simulink model "roboticArm"  (R2021a)
settings: Solver=FixedStepDiscrete  StartTime=0.0  StopTime=inf  FixedStep=0.001  RelTol=1e-3  EnableMultiTasking=on
PreLoadFcn:
  | set_param(gcs, 'RTWSystemTargetFile', 'franka_emika_panda.tlc');%
  | %initRoboticArm();
values from neighbouring files (symbols this model uses):
  amp = 0.05*100    (= 5)    [initRoboticArm.m]    (also in initRoboticArm2.m = 0.5)
  dof = 1    [initRoboticArm.m]    (also in initRoboticArm2.m)
  init_delay = 10    [initRoboticArm.m]    (also in initRoboticArm2.m)
  Kd_matr = zeros(6)    [initRoboticArm.m]    (also in init_roboticArm_loadCell.m = diag([0.00;0;0.003;0.0001;0.00;0.0001]); zeroForce2.mat = [0 0 0 0 0 0 0 0 0 0 0 0 ... (36 elements, 6x6)])
  Ki_matr = zeros(6)    [initRoboticArm.m]    (also in init_roboticArm_loadCell.m = diag([10;100;10;30;10;2]); zeroForce2.mat = [10 0 0 0 0 0 0 100 0 0 0 0 ... (36 elements, 6x6)])
  Kp_matr = zeros(6)    [initRoboticArm.m]    (also in init_roboticArm_loadCell.m = diag([0.3;0.1;0.2;0.05;0.3;0.2]); zeroForce2.mat = [0.3 0 0 0 0 0 0 0.1 0 0 0 0 ... (36 elements, 6x6)])
  scaled_array = zeros(round((chirp_duration+10)*1./dt-1)+1,7)    [initRoboticArm.m]    (also in init_roboticArm_loadCell.m = [scaled_array(:,1) zeros(length(scaled_array),6)]; scaled_array_oc5.mat = [0 0.0141421356237 0.0282842712475 0.0424264068712 0.0565685; zeroForce2.mat = [0 0.0141421356237 0.0282842712475 0.0424264068712 0.0565685)
  tuning_signal = 2    [initRoboticArm.m]    (also in initRoboticArm2.m = 4)
undefined symbols (not defined in the file or in its folder): DiscIntNeverNeededParam
libraries: spsSampleandHoldLib x12, franka_simulink_library x5, simulink x3, etargetslib x1, dspnetwork x1
settings Model: ExtModeTrigDuration=10000  Creator=vasi_ko  LastModifiedBy=host
settings SolverCC: AlgebraicLoopSolver=TrustRegion
settings DataIOCC: SaveFormat=Array  ReturnWorkspaceOutputs=off
settings OptimizationCC: DefaultParameterBehavior=Inlined  EnhancedBackFolding=on  PassReuseOutputArgsThreshold=0  OptimizeBlockOrder=speed  DifferentSizesBufferReuse=on  OptimizationCustomize=off
settings DebuggingCC: SolverPrmCheckMsg=warning  ParameterTunabilityLossMsg=error  SFUnexpectedBacktrackingDiag=warning  SFNoUnconditionalDefaultTransitionDiag=warning  SFExecutionAtInitializationDiag=none  SFMachineParentedDataDiag=warning  ArithmeticOperatorsInVariantConditions=warning
settings HardwareCC: ProdBitPerLong=64  ProdHWDeviceType=Intel->x86-64 (Linux 64)
settings ModelReferenceCC: PropagateSignalLabelsOutOfModel=off
settings SFSimCC: SimUseLocalCustomCode=off  MATLABDynamicMemAlloc=off  CustomCodeUndefinedFunction=UseInterfaceOnly  SimTargetLang=C++
settings RTWCC: Description=Generic Real-Time Target  SystemTargetFile=franka_emika_panda.tlc  RTWVerbose=off  RTWUseLocalCustomCode=off  Toolchain=Franka Simulink | gmake (64-bit linux)  BuildConfiguration=Faster Runs  TargetLang=C++
settings CodeAppCC: ForceParamTrailComments=on  OperatorAnnotations=on
settings STFCustomTargetCC: TargetLangStandard=C99 (ISO)  ModelReferenceCompliant=off  MatFileLogging=on  SystemTargetFile=franka_emika_panda.tlc
settings GRTTargetCC: ModelReferenceCompliant=off  ParMdlRefBuildCompliant=off  CompOptLevelCompliant=off  ConcurrentExecutionCompliant=off  CombineOutputUpdateFcns=off  CPPClassGenCompliant=off  GRTInterface=on  ExtModeStaticAlloc=on  ExtModeTransport=1  ExtModeMexFile=ext_xcp  ExtModeIntrfLevel=Level2 - Open
settings ConfigComp: CovMetricSettings=dw  CovSaveCumulativeToWorkspaceVar=on  CovSaveSingleToWorkspaceVar=on  CovExternalEMLEnable=off  CovSFcnEnable=off

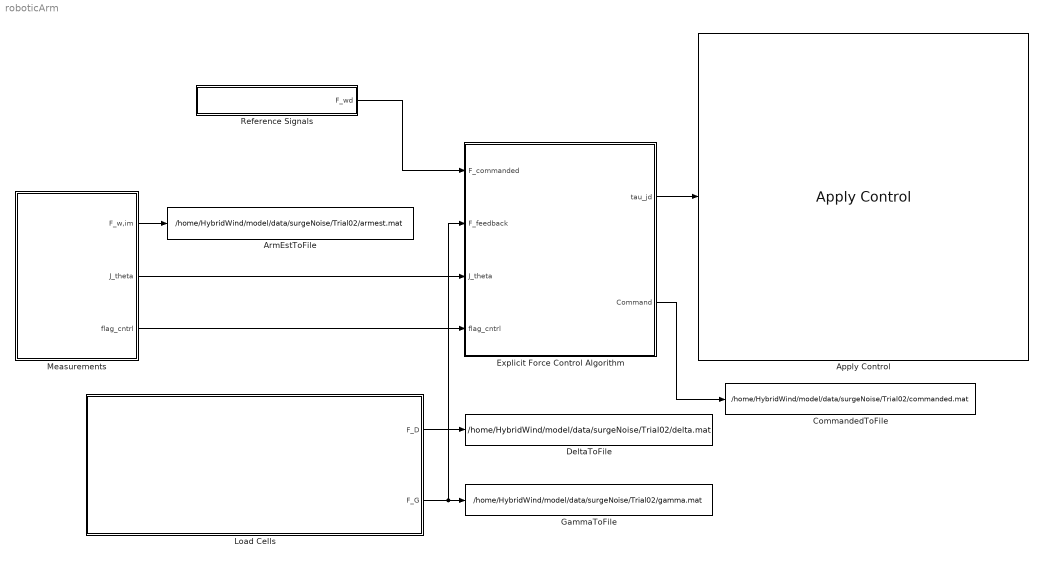
== system roboticArm ==
  Apply Control : franka_simulink_library/Apply Control  robot_ip=robot_ip  gripper_attached=off  control_mode=Torque Control  controller_choice=Joint Impedance Controller  elbow_control=on  collision_thresholds=100*ones(1,52)  joint_impedance=joint_impedance  cartesian_impedance=cartesian_impedance  load_inertia=load_inertia  EE_T_K=EE_T_K  init_joint_configuration_req=off  init_joint_configuration=[0.00392584915725334;-0.104076810189763;0.0404703493577216;-2.7334242600631;0.0113035300040543;2.63364770337236;0.372162046953987]
      settings: SourceProductName=Franka Emika
  ArmEstToFile : ToFile  Filename=/home/HybridWind/model/data/surgeNoise/Trial02/armest.mat  MatrixName=armest
  CommandedToFile : ToFile  Filename=/home/HybridWind/model/data/surgeNoise/Trial02/commanded.mat  MatrixName=commanded
  DeltaToFile : ToFile  Filename=/home/HybridWind/model/data/surgeNoise/Trial02/delta.mat  MatrixName=delta
  Explicit Force Control Algorithm : Subsystem
  GammaToFile : ToFile  Filename=/home/HybridWind/model/data/surgeNoise/Trial02/gamma.mat  MatrixName=gamma
  Load Cells : Subsystem
  Measurements : Subsystem
  Reference Signals : Subsystem
  wires:
  Measurements/3(flag_cntrl) -> Explicit Force Control Algorithm/4(flag_cntrl)
  Load Cells/2(F_G) -> Explicit Force Control Algorithm/2(F_feedback), GammaToFile/1
  Explicit Force Control Algorithm/1(tau_jd) -> Apply Control/1
  Reference Signals/1(F_wd) -> Explicit Force Control Algorithm/1(F_commanded)
  Measurements/2(J_theta) -> Explicit Force Control Algorithm/3(J_theta)
  Measurements/1(F_w,im) -> ArmEstToFile/1
  Explicit Force Control Algorithm/2(Command) -> CommandedToFile/1
  Load Cells/1(F_D) -> DeltaToFile/1

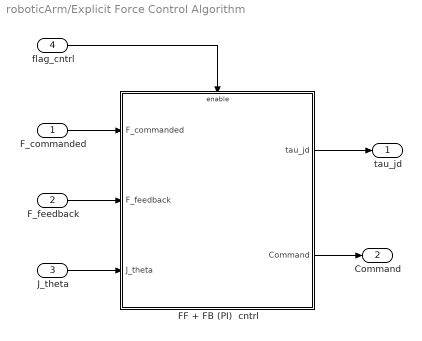
== system roboticArm/Explicit Force Control Algorithm ==
  F_commanded : Inport
  F_feedback : Inport  Port=2
  J_theta : Inport  Port=3
  flag_cntrl : Inport  Port=4
  FF + FB (PI)  cntrl : Subsystem
  tau_jd : Outport
  Command : Outport  Port=2
  wires:
  F_commanded/1 -> FF + FB (PI)  cntrl/1(F_commanded)
  F_feedback/1 -> FF + FB (PI)  cntrl/2(F_feedback)
  J_theta/1 -> FF + FB (PI)  cntrl/3(J_theta)
  FF + FB (PI)  cntrl/1(tau_jd) -> tau_jd/1
  flag_cntrl/1 -> FF + FB (PI)  cntrl/Enable
  FF + FB (PI)  cntrl/2(Command) -> Command/1

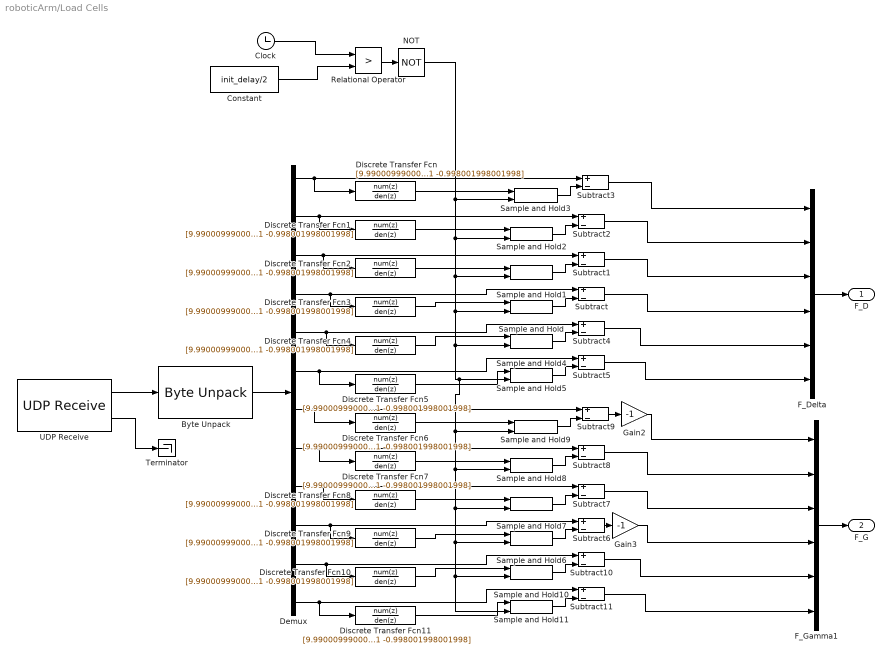
== system roboticArm/Load Cells ==
  Byte Unpack : etargetslib/Byte Unpack  dimensions={[12]}  datatypes={'double'}  byteAlign=1
  Clock : Clock
  Constant : Constant  Value=init_delay/2
  Demux : Demux  Outputs=12
  Discrete Transfer Fcn{,1..11} (12 alike) : DiscreteTransferFcn  Numerator=[9.990009990009990e-04 9.990009990009990e-04]  Denominator=[1 -0.998001998001998]
  F_Delta : Mux  Inputs=6
  F_Gamma1 : Mux  Inputs=6
  Gain2 : Gain  Gain=-1
  Gain3 : Gain  Gain=-1
  NOT : Logic  Operator=NOT  IconShape=distinctive  AllPortsSameDT=off  OutDataTypeStr=boolean
  Relational Operator : RelationalOperator  Operator=>  OutDataTypeStr=boolean  RndMeth=Simplest
  Sample and Hold{,1..11} (12 alike) : spsSampleandHoldLib/Sample and Hold  ic=0  Ts=0
      settings: SourceProductBaseCode=PS
  Subtract{,1..11} (12 alike) : Sum  Inputs=+-
  Terminator : Terminator
  UDP Receive : dspnetwork/UDP Receive  localURL='0.0.0.0'  localPort=8002  remoteURL='10.10.10.15'  remotePort=-1  recvBufferSize=8192  dims=96  signalDatatype=uint8  isComplex=off  isVarSize=off  showBlockingTime=on  blockingTime=inf  sampletime=0.001  blockPlatform=HOST
  F_D : Outport
  F_G : Outport  Port=2
  wires:
  UDP Receive/1 -> Byte Unpack/1
  Constant/1 -> Relational Operator/2
  Relational Operator/1 -> NOT/1
  Sample and Hold/1 -> Subtract/2
  UDP Receive/2 -> Terminator/1
  Demux/4 -> Discrete Transfer Fcn3/1, Subtract/1
  Clock/1 -> Relational Operator/1
  Byte Unpack/1 -> Demux/1
  Demux/3 -> Discrete Transfer Fcn2/1, Subtract1/1
  Sample and Hold1/1 -> Subtract1/2
  Subtract1/1 -> F_Delta/3
  Subtract2/1 -> F_Delta/2
  Sample and Hold2/1 -> Subtract2/2
  Demux/2 -> Discrete Transfer Fcn1/1, Subtract2/1
  Sample and Hold3/1 -> Subtract3/2
  Subtract4/1 -> F_Delta/5
  Sample and Hold4/1 -> Subtract4/2
  Demux/5 -> Discrete Transfer Fcn4/1, Subtract4/1
  Demux/6 -> Discrete Transfer Fcn5/1, Subtract5/1
  Sample and Hold5/1 -> Subtract5/2
  Subtract5/1 -> F_Delta/6
  Subtract3/1 -> F_Delta/1
  Subtract/1 -> F_Delta/4
  F_Delta/1 -> F_D/1
  Demux/1 -> Discrete Transfer Fcn/1, Subtract3/1
  Discrete Transfer Fcn/1 -> Sample and Hold3/1
  Discrete Transfer Fcn1/1 -> Sample and Hold2/1
  Discrete Transfer Fcn2/1 -> Sample and Hold1/1
  Discrete Transfer Fcn3/1 -> Sample and Hold/1
  Discrete Transfer Fcn4/1 -> Sample and Hold4/1
  Discrete Transfer Fcn5/1 -> Sample and Hold5/1
  Discrete Transfer Fcn11/1 -> Sample and Hold11/1
  Discrete Transfer Fcn10/1 -> Sample and Hold10/1
  Discrete Transfer Fcn9/1 -> Sample and Hold6/1
  Discrete Transfer Fcn8/1 -> Sample and Hold7/1
  Discrete Transfer Fcn7/1 -> Sample and Hold8/1
  Discrete Transfer Fcn6/1 -> Sample and Hold9/1
  Demux/7 -> Subtract9/1, Discrete Transfer Fcn6/1
  F_Gamma1/1 -> F_G/1
  Gain3/1 -> F_Gamma1/4
  Gain2/1 -> F_Gamma1/1
  Subtract11/1 -> F_Gamma1/6
  Sample and Hold11/1 -> Subtract11/2
  NOT/1 -> Sample and Hold3/2, Sample and Hold2/2, Sample and Hold1/2, Sample and Hold6/2, Sample and Hold10/2, Sample and Hold11/2, Sample and Hold7/2, Sample and Hold8/2, Sample and Hold9/2, Sample and Hold5/2, Sample and Hold4/2, Sample and Hold/2
  Demux/12 -> Subtract11/1, Discrete Transfer Fcn11/1
  Demux/11 -> Subtract10/1, Discrete Transfer Fcn10/1
  Sample and Hold10/1 -> Subtract10/2
  Subtract10/1 -> F_Gamma1/5
  Subtract9/1 -> Gain2/1
  Sample and Hold9/1 -> Subtract9/2
  Demux/8 -> Subtract8/1, Discrete Transfer Fcn7/1
  Sample and Hold8/1 -> Subtract8/2
  Subtract8/1 -> F_Gamma1/2
  Subtract7/1 -> F_Gamma1/3
  Sample and Hold7/1 -> Subtract7/2
  Demux/9 -> Subtract7/1, Discrete Transfer Fcn8/1
  Demux/10 -> Subtract6/1, Discrete Transfer Fcn9/1
  Sample and Hold6/1 -> Subtract6/2
  Subtract6/1 -> Gain3/1

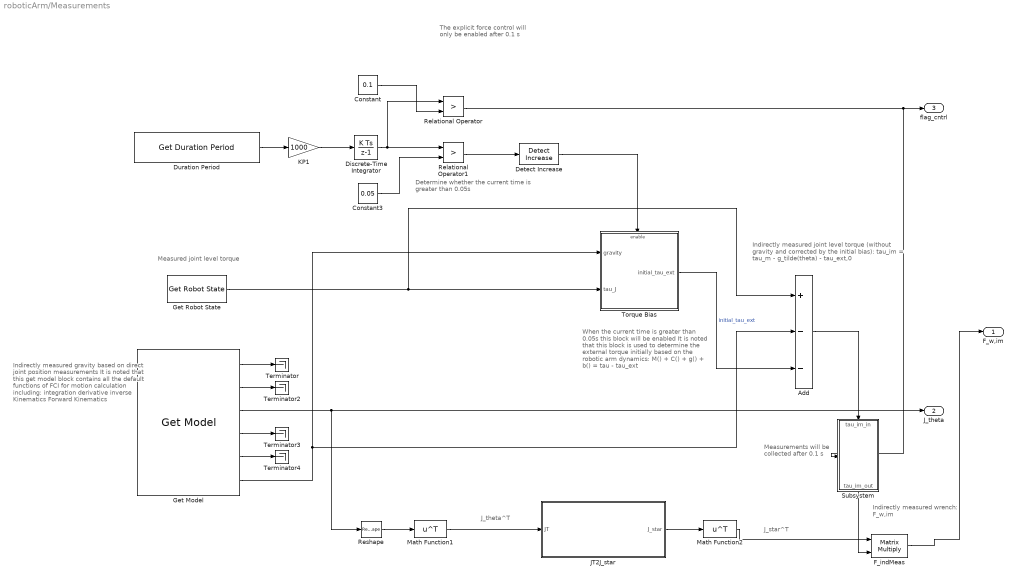
== system roboticArm/Measurements ==
  note: Indirectly measured wrench:
      | F_w,im
  note: J_star^T
  note: J_theta^T
  note: The explicit force control will only be enabled after 0.1 s
  note: When the current time is greater than 0.05s this block will be enabled
      |
      | It is noted that this block is used to determine the external torque initially based on the robotic arm dynamics:
      |
      | M() + C() + g() + b() = tau - tau_ext
  note: Determine whether the current time is greater than 0.05s
  note: Measured joint level torque
  note: Indirectly measured gravity based on direct joint position measurements
      |
      | It is noted that this get model block contains all the default functions of FCI for motion calculation including:
      | integration
      | derivative
      | inverse Kinematics
      | Forward Kinematics
  note: Indirectly measured joint level torque (without gravity and corrected by the initial bias):
      | tau_im = tau_m - g_tilde(theta) - tau_ext,0
  note: Measurements will be collected after 0.1 s
  Add : Sum  Inputs=+--
  Constant : Constant  Value=0.1
  Constant3 : Constant  Value=0.05
  Detect Increase : simulink/Logic and Bit Operations/Detect Increase  vinit=0.0  OutDataTypeStr=boolean
  Discrete-Time Integrator : DiscreteIntegrator  SampleTime=-1  ICPrevOutput=DiscIntNeverNeededParam  ICPrevScaledInput=DiscIntNeverNeededParam
  Duration Period : franka_simulink_library/Get Duration Period  robot_ip=robot_ip
      settings: SourceProductName=Franka Emika
  F_indMeas : Product  Multiplication=Matrix(*)
  Get Model : franka_simulink_library/Get Model  robot_ip=robot_ip
      settings: SourceProductName=Franka Emika
  Get Robot State : franka_simulink_library/Get Robot State  robot_ip=robot_ip  signals_requested='tau_J'
      settings: SourceProductName=Franka Emika
  JT2J_star : MATLAB Function  TreatAsAtomicUnit=on
  KP1 : Gain  Gain=1000
  Math Function1 : Math  Operator=transpose  SignedPower=on  SaturateOnIntegerOverflow=on
  Math Function2 : Math  Operator=transpose  SignedPower=on  SaturateOnIntegerOverflow=on
  Relational Operator : RelationalOperator  Operator=>  OutDataTypeStr=boolean  RndMeth=Nearest
  Relational Operator1 : RelationalOperator  Operator=>  OutDataTypeStr=boolean  RndMeth=Nearest
  Reshape : Reshape  OutputDimensionality=Customize  OutputDimensions=[6,7]
  Subsystem : Subsystem
  Terminator{,2..4} (4 alike) : Terminator
  Torque Bias : Subsystem
  F_w,im : Outport
  J_theta : Outport  Port=2
  flag_cntrl : Outport  Port=3
  wires:
  Relational Operator1/1 -> Detect Increase/1
  Duration Period/1 -> KP1/1
  Constant3/1 -> Relational Operator1/2
  Discrete-Time Integrator/1 -> Relational Operator/1, Relational Operator1/1
  KP1/1 -> Discrete-Time Integrator/1
  Detect Increase/1 -> Torque Bias/Enable
  Get Robot State/1 -> Add/1, Torque Bias/2(tau_J)
  Get Model/6 -> Add/2, Torque Bias/1(gravity)
  Get Model/1 -> Terminator/1
  Get Model/2 -> Terminator2/1
  Get Model/4 -> Terminator3/1
  Get Model/5 -> Terminator4/1
  Torque Bias/1(initial_tau_ext) -> Add/3  "initial_tau_ext"
  Add/1 -> Subsystem/1(tau_im_in)
  Get Model/3 -> Reshape/1, J_theta/1
  Reshape/1 -> Math Function1/1
  Math Function1/1 -> JT2J_star/1(JT)
  JT2J_star/1(J_star) -> Math Function2/1
  Math Function2/1 -> F_indMeas/1
  F_indMeas/1 -> F_w,im/1
  Constant/1 -> Relational Operator/2
  Relational Operator/1 -> Subsystem/Enable, flag_cntrl/1
  Subsystem/1(tau_im_out) -> F_indMeas/2

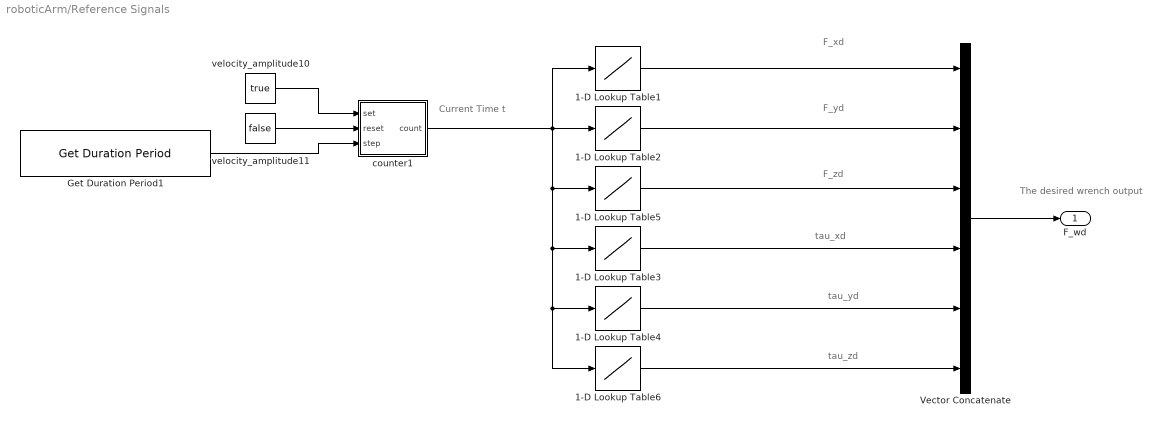
== system roboticArm/Reference Signals ==
  note: Current Time t
  note: F_xd
  note: F_yd
  note: F_zd
  note: tau_xd
  note: tau_yd
  note: tau_zd
  note: The desired wrench output
  1-D Lookup Table1 : Lookup_n-D  NumberOfTableDimensions=1  BreakpointsForDimension1=scaled_array(:,1)  Table=scaled_array(:,2)  InternalRulePriority=Speed  RndMeth=Simplest  InputSameDT=on
  1-D Lookup Table2 : Lookup_n-D  NumberOfTableDimensions=1  BreakpointsForDimension1=scaled_array(:,1)  Table=scaled_array(:,3)  InternalRulePriority=Speed  RndMeth=Simplest  InputSameDT=on
  1-D Lookup Table3 : Lookup_n-D  NumberOfTableDimensions=1  BreakpointsForDimension1=scaled_array(:,1)  Table=scaled_array(:,5)  InternalRulePriority=Speed  RndMeth=Simplest  InputSameDT=on
  1-D Lookup Table4 : Lookup_n-D  NumberOfTableDimensions=1  BreakpointsForDimension1=scaled_array(:,1)  Table=scaled_array(:,6)  InternalRulePriority=Speed  RndMeth=Simplest  InputSameDT=on
  1-D Lookup Table5 : Lookup_n-D  NumberOfTableDimensions=1  BreakpointsForDimension1=scaled_array(:,1)  Table=scaled_array(:,4)  InternalRulePriority=Speed  RndMeth=Simplest  InputSameDT=on
  1-D Lookup Table6 : Lookup_n-D  NumberOfTableDimensions=1  BreakpointsForDimension1=scaled_array(:,1)  Table=scaled_array(:,7)  InternalRulePriority=Speed  RndMeth=Simplest  InputSameDT=on
  Get Duration Period1 : franka_simulink_library/Get Duration Period  robot_ip=robot_ip
      settings: SourceProductName=Franka Emika
  Vector Concatenate : Concatenate  NumInputs=6
  counter1 : Subsystem
  velocity_amplitude10 : Constant  Value=true  VectorParams1D=off
  velocity_amplitude11 : Constant  Value=false  VectorParams1D=off
  F_wd : Outport
  wires:
  counter1/1(count) -> 1-D Lookup Table6/1, 1-D Lookup Table4/1, 1-D Lookup Table3/1, 1-D Lookup Table5/1, 1-D Lookup Table2/1, 1-D Lookup Table1/1
  Vector Concatenate/1 -> F_wd/1
  Get Duration Period1/1 -> counter1/3(step)
  velocity_amplitude10/1 -> counter1/1(set)
  velocity_amplitude11/1 -> counter1/2(reset)
  1-D Lookup Table5/1 -> Vector Concatenate/3
  1-D Lookup Table3/1 -> Vector Concatenate/4
  1-D Lookup Table6/1 -> Vector Concatenate/6
  1-D Lookup Table4/1 -> Vector Concatenate/5
  1-D Lookup Table1/1 -> Vector Concatenate/1
  1-D Lookup Table2/1 -> Vector Concatenate/2

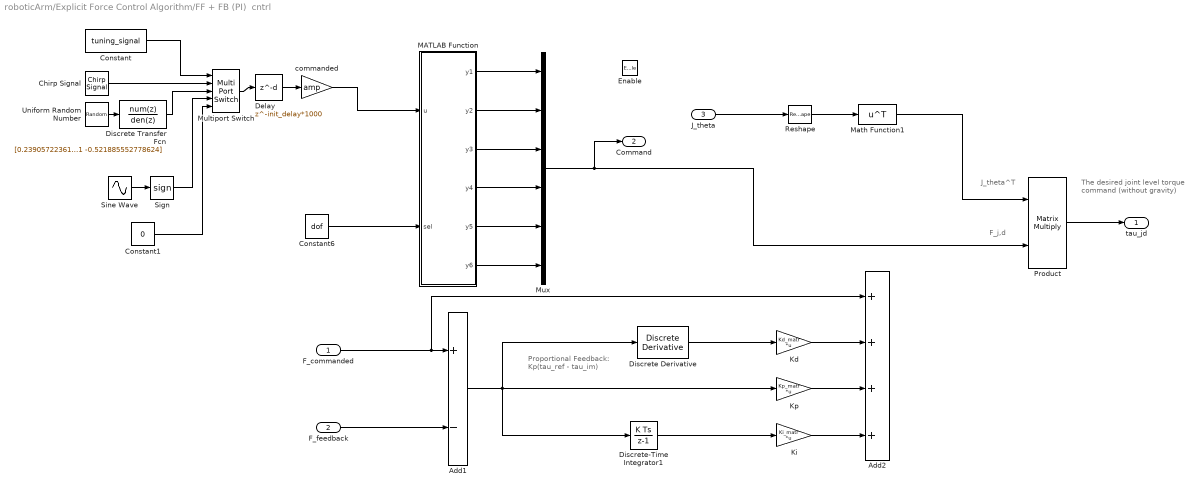
== system roboticArm/Explicit Force Control Algorithm/FF + FB (PI)  cntrl ==
  note: F_j,d
  note: The desired joint level torque command (without gravity)
  note: Proportional Feedback:
      |  Kp(tau_ref - tau_im)
  note: J_theta^T
  F_commanded : Inport
  F_feedback : Inport  Port=2
  J_theta : Inport  Port=3
  Enable : EnablePort
  Add1 : Sum  Inputs=+-
  Add2 : Sum  Inputs=++++
  Chirp Signal : simulink/Sources/Chirp Signal  f1=0.1  T=60  f2=20
  Constant : Constant  Value=tuning_signal
  Constant1 : Constant  Value=0
  Constant6 : Constant  Value=dof
  Delay : Delay  DelayLength=init_delay*1000
  Discrete Transfer Fcn : DiscreteTransferFcn  Numerator=[0.239057223610688 0.239057223610688]  Denominator=[1 -0.521885552778624]
  Discrete Derivative : simulink/Discrete/Discrete Derivative  gainval=1.0  ICPrevScaledInput=0.0  OutMin=[]  OutMax=[]  OutDataType=fixdt(1, 16)  OutScaling=2^-10  DoSatur=off
  Discrete-Time Integrator1 : DiscreteIntegrator  SampleTime=0.001  ICPrevOutput=DiscIntNeverNeededParam  ICPrevScaledInput=DiscIntNeverNeededParam
  Kd : Gain  Gain=Kd_matr  Multiplication=Matrix(K*u)
  Ki : Gain  Gain=Ki_matr  Multiplication=Matrix(K*u)
  Kp : Gain  Gain=Kp_matr  Multiplication=Matrix(K*u)
  MATLAB Function : MATLAB Function  TreatAsAtomicUnit=on
  Math Function1 : Math  Operator=transpose  SignedPower=on  SaturateOnIntegerOverflow=on
  Multiport Switch : MultiPortSwitch  Inputs=4
  Mux : Mux  Inputs=6
  Product : Product  Multiplication=Matrix(*)
  Reshape : Reshape  OutputDimensionality=Customize  OutputDimensions=[6,7]
  Sign : Signum
  Sine Wave : Sin  Frequency=2*pi/60  SampleTime=0
  Uniform Random Number : UniformRandomNumber  SampleTime=0.001
  commanded : Gain  Gain=amp
  tau_jd : Outport
  Command : Outport  Port=2
  wires:
  Add1/1 -> Discrete Derivative/1, Discrete-Time Integrator1/1, Kp/1
  F_commanded/1 -> Add2/1, Add1/1
  Reshape/1 -> Math Function1/1
  J_theta/1 -> Reshape/1
  Math Function1/1 -> Product/1
  Discrete-Time Integrator1/1 -> Ki/1
  Discrete Derivative/1 -> Kd/1
  Kp/1 -> Add2/3
  Ki/1 -> Add2/4
  Kd/1 -> Add2/2
  F_feedback/1 -> Add1/2
  Product/1 -> tau_jd/1
  Mux/1 -> Command/1, Product/2
  Uniform Random Number/1 -> Discrete Transfer Fcn/1
  commanded/1 -> MATLAB Function/1(u)
  Constant6/1 -> MATLAB Function/2(sel)
  MATLAB Function/1(y1) -> Mux/1
  MATLAB Function/2(y2) -> Mux/2
  MATLAB Function/3(y3) -> Mux/3
  MATLAB Function/4(y4) -> Mux/4
  MATLAB Function/5(y5) -> Mux/5
  MATLAB Function/6(y6) -> Mux/6
  Delay/1 -> commanded/1
  Chirp Signal/1 -> Multiport Switch/2
  Discrete Transfer Fcn/1 -> Multiport Switch/3
  Constant/1 -> Multiport Switch/1
  Multiport Switch/1 -> Delay/1
  Sine Wave/1 -> Sign/1
  Sign/1 -> Multiport Switch/4
  Constant1/1 -> Multiport Switch/5

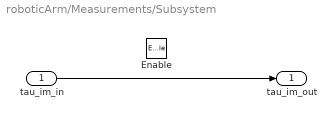
== system roboticArm/Measurements/Subsystem ==
  tau_im_in : Inport
  Enable : EnablePort
  tau_im_out : Outport
  wires:
  tau_im_in/1 -> tau_im_out/1

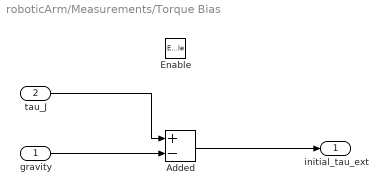
== system roboticArm/Measurements/Torque Bias ==
  gravity : Inport
  tau_J : Inport  Port=2
  Enable : EnablePort
  Added : Sum  Inputs=+-
  initial_tau_ext : Outport  InitialOutput=[0 0 0 0 0 0 0]  VectorParamsAs1DForOutWhenUnconnected=off
  wires:
  tau_J/1 -> Added/1
  gravity/1 -> Added/2
  Added/1 -> initial_tau_ext/1

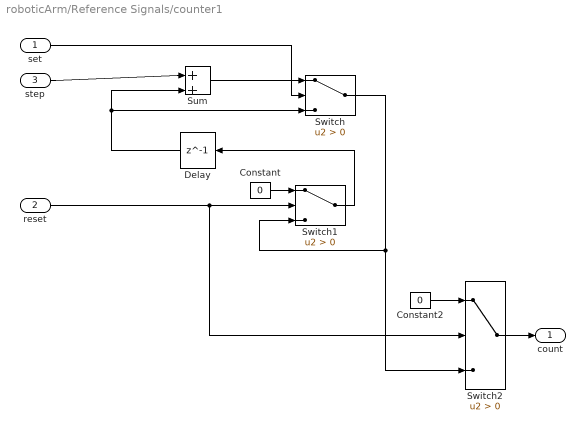
== system roboticArm/Reference Signals/counter1 ==
  set : Inport  OutDataTypeStr=boolean
  reset : Inport  Port=2  OutDataTypeStr=boolean
  step : Inport  Port=3  OutDataTypeStr=double
  Constant : Constant  Value=0  OutDataTypeStr=double
  Constant2 : Constant  Value=0  OutDataTypeStr=double
  Delay : Delay  DelayLength=1  InitialCondition=0
  Sum : Sum  Inputs=|++
  Switch : Switch  Criteria=u2 > Threshold
  Switch1 : Switch  Criteria=u2 > Threshold  OutDataTypeStr=double
  Switch2 : Switch  Criteria=u2 > Threshold  OutDataTypeStr=double
  count : Outport  OutDataTypeStr=double  VectorParamsAs1DForOutWhenUnconnected=off
  wires:
  Switch2/1 -> count/1
  Constant2/1 -> Switch2/1
  Sum/1 -> Switch/1
  set/1 -> Switch/2
  Switch/1 -> Switch1/3, Switch2/3
  step/1 -> Sum/1
  Delay/1 -> Sum/2, Switch/3
  reset/1 -> Switch1/2, Switch2/2
  Constant/1 -> Switch1/1
  Switch1/1 -> Delay/1

== matlab function roboticArm/Explicit Force Control Algorithm/FF + FB (PI)  cntrl/MATLAB Function ==
  data: u input; y1 output; sel input; y2 output; y3 output; y4 output; y5 output; y6 output
function [y1, y2, y3, y4, y5, y6] = fcn(u, sel)

y1 = 0;
y2 = 0;
y3 = 0;
y4 = 0;
y5 = 0;
y6 = 0;

switch sel
    case 1
        y1 = u;
    case 2
        y2 = u;
    case 3
        y3 = u;
    case 4
        y4 = u;
    case 5
        y5 = u;
    case 6
        y6 = u;
    otherwise
        y1 = 0;
end

== matlab function roboticArm/Measurements/JT2J_star ==
  data: JT input; J_star output
function J_star = JT2J_star(JT)
%#codegen

J = JT';
% low isotropic damping, the value should be much smaller than lambda_max^2
beta =0;
% damping added in singular directions, we chose it to be equal to
% threshold
% lambda_max = singularity_threshold_inverse_kinematics; 
% SVD decomposition
[U,S,~] = svd(J);
sigma = diag(S);
% rank
singularity_threshold_inverse_kinematics = eps;
r = sum(sigma > singularity_threshold_inverse_kinematics);
% initilizing damping
  lambda_square_vector = zeros(6,1);
if r==6 % damping in full rank case is zero
    lambda_square_vector = zeros(6,1);
else % daamping in rank deficient cases
%     sigma_singular = sigma(r+1:6);
%     lambda_square_vector(r+1:6) = ...
%         (1 - (sigma_singular/ singularity_threshold_inverse_kinematics).^2) *...
%         lambda_max^2;
end
J_star =  JT * U * diag(1./(sigma.^2+lambda_square_vector+beta^2*ones(6,1)))*U';

end
